simulink model "ss_feedback_simulink"  (R2022b)
settings: Solver=VariableStepAuto  StartTime=0.0  StopTime=10.0  RelTol=1e-3
libraries: MainLibrary x1
settings Model: Creator=cotti  LastModifiedBy=cotti

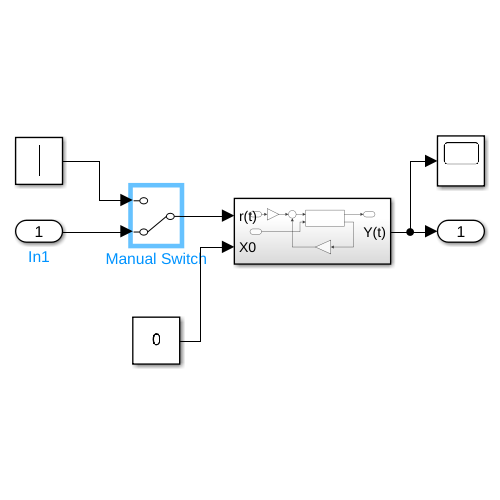
[thumbnail: Simulink's stored preview of the top-level diagram]
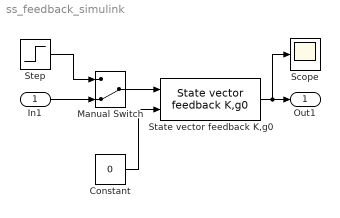
== system ss_feedback_simulink ==
  In1 : Inport
  Constant : Constant  Value=0
  Manual Switch : ManualSwitch  CurrentSetting=0
  Scope : Scope
  State vector feedback K,g0 : MainLibrary/State vector feedback K,g0  SystemSampleTime=-1  VariantActivationTime=update diagram  Latency=0  AutoFrameSizeCalculation=off
  Step : Step  SampleTime=0
  Out1 : Outport
  wires:
  State vector feedback K,g0/1 -> Scope/1, Out1/1
  Constant/1 -> State vector feedback K,g0/2
  In1/1 -> Manual Switch/2
  Manual Switch/1 -> State vector feedback K,g0/1
  Step/1 -> Manual Switch/1
